simulink model "BimanualHD2LfD"  (R2016b)
settings: Solver=ode1  StartTime=0.0  StopTime=inf  FixedStep=0.002  RelTol=1e-3  EnableMultiTasking=on
undefined symbols (not defined in the file or in its folder): d2r, HIL, qc_get_step_size
libraries: quarc_library x10, simulink_extras x4, dsparch4 x3, simulink x2
(part 1 of 2)
settings Model: SimulationMode=external  ExtModeTrigDuration=120000  Creator=user  LastModifiedBy=Jason
settings SolverCC: PositivePriorityOrder=on
settings DataIOCC: LimitDataPoints=on  SaveFormat=Array  SignalLoggingSaveFormat=ModelDataLogs
settings OptimizationCC: ExpressionDepthLimit=2147483647  LifeSpan=inf
settings DebuggingCC: UnderspecifiedInitializationDetection=Classic  MergeDetectMultiDrivingBlocksExec=none  SolverPrmCheckMsg=warning  FcnCallInpInsideContextMsg=warning  StateNameClashWarn=warning  SFUnexpectedBacktrackingDiag=warning  SFNoUnconditionalDefaultTransitionDiag=warning  SFExecutionAtInitializationDiag=none
settings HardwareCC: ProdBitPerPointer=32  ProdBitPerSizeT=32  ProdBitPerPtrDiffT=32  ProdLargestAtomicFloat=None  ProdIntDivRoundTo=Undefined  ProdEndianess=Unspecified  ProdWordSize=32  ProdHWDeviceType=32-bit Generic
settings ModelReferenceCC: PropagateSignalLabelsOutOfModel=off
settings RTWCC: SystemTargetFile=quarc_windows.tlc  TemplateMakefile=quarc_default_tmf  Description=QUARC Win32 Target
settings STFCustomTargetCC: TargetPreCompLibLocation=C:\PROGRA~2\QUARC\lib\2011b\windows\release  GeneratePreprocessorConditionals=Disable all  CPPClassGenCompliant=on  SystemTargetFile=quarc_windows.tlc
settings GRTTargetCC: TargetPreCompLibLocation=C:\PROGRA~2\QUARC\lib\2011b\windows\release  TargetLangStandard=C89/C90 (ANSI)  ParMdlRefBuildCompliant=off  CompOptLevelCompliant=off  ConcurrentExecutionCompliant=off  GeneratePreprocessorConditionals=Disable all  CombineOutputUpdateFcns=off  MatFileLogging=off  GRTInterface=on  UseToolchainInfoCompliant=off  ExtMode=on  ExtModeMexFile=quarc_comm
settings ConfigComp: CovMetricSettings=dw  CovHtmlReporting=on  CovSaveCumulativeToWorkspaceVar=on  CovSaveSingleToWorkspaceVar=on  CovExternalEMLEnable=off
settings SimEventsCC: propDiagStatOutput=1  propPreventDuplicateEvents=0

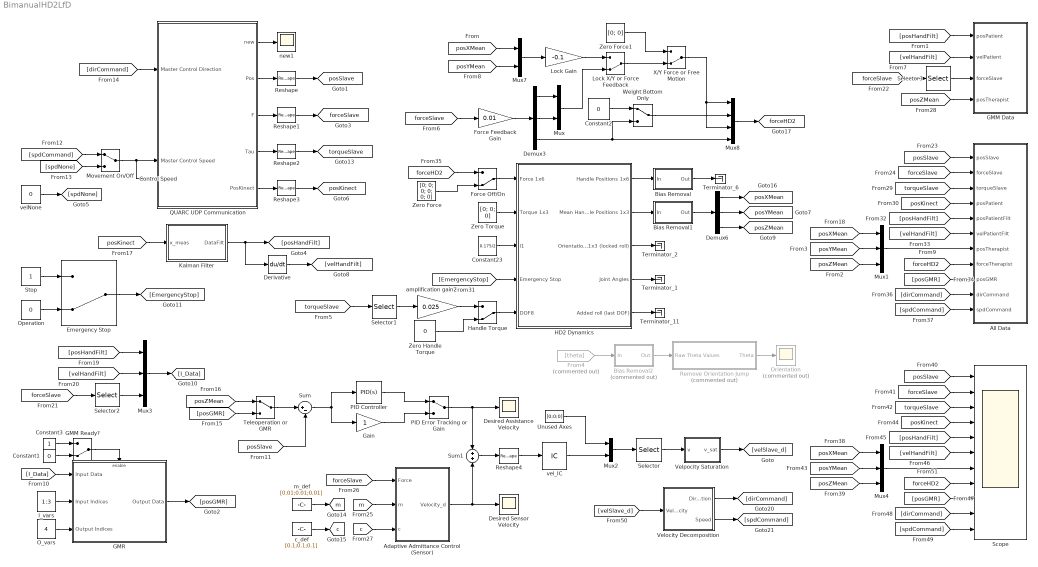
== system BimanualHD2LfD ==
  Adaptive Admittance Control (Sensor) : Subsystem
  All Data : Subsystem  TreatAsAtomicUnit=on
  Bias Removal : Subsystem
  Bias Removal1 : Subsystem
  Bias Removal2 : Subsystem  Commented=on
  Constant1 : Constant  Value=0
  Constant2 : Constant  Value=0
  Constant23 : Constant  Value=0.175/2
  Constant3 : Constant
  Control Speed : Scope
  Demux3 : Demux  Outputs=3
  Demux6 : Demux  Outputs=3
  Derivative : Derivative
  Desired Assistance Velocity : Scope
  Desired Sensor Velocity : Scope
  Emergency Stop : ManualSwitch  CurrentSetting=0
  Force Feedback Gain : Gain  Gain=0.01
  Force Off/On : ManualSwitch  CurrentSetting=0
  From4 : From  Commented=on  GotoTag=theta  TagVisibility=global
  GMM Data : Subsystem  TreatAsAtomicUnit=on
  GMM Ready? : ManualSwitch  CurrentSetting=0
  GMR : Subsystem
  Gain : Gain
  HD2 Dynamics : Subsystem
  Handle Torque : ManualSwitch  CurrentSetting=0
  I_vars : Constant  Value=1:3
  Kalman Filter : MATLAB Function  TreatAsAtomicUnit=on
  Lock Gain : Gain  Gain=-0.1
  Lock X/Y or Force Feedback : ManualSwitch  CurrentSetting=0
  Movement On/Off : ManualSwitch
  Mux : Mux  Inputs=2
  Mux1 : Mux  Inputs=3
  Mux2 : Mux  Inputs=2
  Mux3 : Mux  Inputs=3
  Mux4 : Mux  Inputs=3
  Mux7 : Mux  Inputs=2
  Mux8 : Mux
  O_vars : Constant  Value=4
  Operation : Constant  Value=0
  Orientation : Scope  Commented=on
  PID Controller : simulink/Continuous/PID Controller  Controller=PID  TimeDomain=Continuous-time  SampleTime=-1  IntegratorMethod=Forward Euler  FilterMethod=Forward Euler  Form=Parallel  UseFilter=on  ControllerParametersSource=internal  P=1  I=1  D=0  N=100  InitialConditionSource=internal  InitialConditionForIntegrator=0  InitialConditionForFilter=0  ExternalReset=none  LimitOutput=off  UpperSaturationLimit=inf  LowerSaturationLimit=-inf  LinearizeAsGain=on  AntiWindupMode=none  Kb=1  TrackingMode=off  Kt=1  PParamMin=[]  PParamMax=[]  IParamMin=[]  IParamMax=[]  DParamMin=[]  DParamMax=[]  NParamMin=[]  NParamMax=[]  KbParamMin=[]  KbParamMax=[]  KtParamMin=[]  KtParamMax=[]  POutMin=[]  POutMax=[]  IOutMin=[]  IOutMax=[]  DOutMin=[]  DOutMax=[]  NOutMin=[]  NOutMax=[]  KbOutMin=[]  KbOutMax=[]  KtOutMin=[]  KtOutMax=[]  IntegratorOutMin=[]  IntegratorOutMax=[]  FilterOutMin=[]  FilterOutMax=[]  SumOutMin=[]  SumOutMax=[]  SumI1OutMin=[]  SumI1OutMax=[]  SumI2OutMin=[]  SumI2OutMax=[]  SumI3OutMin=[]  SumI3OutMax=[]  SumDOutMin=[]  SumDOutMax=[]  SaturationOutMin=[]  SaturationOutMax=[]  IntegratorContinuousStateAttributes=''  IntegratorStateMustResolveToSignalObject=off  IntegratorRTWStateStorageClass=Auto  FilterContinuousStateAttributes=''  FilterStateMustResolveToSignalObject=off  FilterRTWStateStorageClass=Auto  DifferentiatorICPrevScaledInput=0  DifferentiatorOutMin=[]  DifferentiatorOutMax=[]
  PID Error Tracking or Gain : ManualSwitch
  QUARC UDP Communication : Subsystem
  Remove Orientation Jump : Subsystem  Commented=on
  Reshape{,1..4} (5 alike) : Reshape  OutputDimensionality=Column vector (2-D)
  Scope : Scope  NumInputPorts=11
  Selector : Selector  InputPortWidth=6  IndexOptions=Index vector (dialog)  Indices=[1 2 6]  OutputSizes=1
  Selector1 : Selector  InputPortWidth=3  IndexOptions=Index vector (dialog)  Indices=[3]  OutputSizes=1
  Selector2 : Selector  InputPortWidth=3  IndexOptions=Index vector (dialog)  Indices=[3]  OutputSizes=1
  Selector3 : Selector  InputPortWidth=3  IndexOptions=Index vector (dialog)  Indices=[3]  OutputSizes=1
  Stop : Constant
  Sum : Sum  Inputs=|+-
  Sum1 : Sum
  Teleoperation or GMR : ManualSwitch
  Terminator_{1..2,6,11} (4 alike) : Terminator
  Unused Axes : Constant  Value=[0;0;0]
  Velocity Decomposition : Subsystem
  Velpocity Saturation : Subsystem
  Weight Bottom Only : ManualSwitch
  X/Y Force or Free Motion : ManualSwitch  CurrentSetting=0
  Zero Force : Constant  Value=[0; 0; 0; 0; 0; 0]
  Zero Force1 : Constant  Value=[0; 0]
  Zero Handle Torque : Constant  Value=0
  Zero Torque : Constant  Value=[0; 0; 0]
  amplification gain2 : Gain  Gain=0.025
  c_def : Constant  Value=[0.1;0.1;0.1]
  m_def : Constant  Value=[0.01;0.01;0.01]
  new1 : Scope
  velNone : Constant  Value=0
  vel_IC : InitialCondition  Value=[0; 0; 0]
  tag scope: c=global, forceHD2=global, forceSlave=global, m=global, posKinect=global, posSlave=global, posXMean=global, posYMean=global, posZMean=global, torqueSlave=global
  wires:
  Zero Torque/1 -> HD2 Dynamics/2(Torque 1x3)
  Constant23/1 -> HD2 Dynamics/3(l1)
  [EmergencyStop] -> HD2 Dynamics/4(Emergency Stop)
  Selector1/1 -> amplification gain2/1
  Handle Torque/1 -> HD2 Dynamics/5(DOF8)
  amplification gain2/1 -> Handle Torque/1
  Zero Handle Torque/1 -> Handle Torque/2
  Demux6/1 -> [posXMean]
  Demux6/2 -> [posYMean]
  Demux6/3 -> [posZMean]
  Force Off/On/1 -> HD2 Dynamics/1(Force 1x6)
  Zero Force/1 -> Force Off/On/2
  HD2 Dynamics/5(Added roll (last DOF)) -> Terminator_11/1
  HD2 Dynamics/4(Joint Angles) -> Terminator_1/1
  HD2 Dynamics/3(Orientation 1x3 (locked roll)) -> Terminator_2/1
  HD2 Dynamics/1(Handle Positions 1x6) -> Bias Removal/1(In)
  Bias Removal/1(Out) -> Terminator_6/1
  [posKinect] -> Kalman Filter/1(x_meas)
  Kalman Filter/1(DataFilt) -> Derivative/1, [posHandFilt]
  HD2 Dynamics/2(Mean Handle Positions 1x3) -> Bias Removal1/1(In)
  Bias Removal1/1(Out) -> Demux6/1
  From4/1 -> Bias Removal2/1(In)
  Bias Removal2/1(Out) -> Remove Orientation Jump/1(Raw Theta Values)
  Remove Orientation Jump/1(Theta) -> Orientation/1
  [forceSlave] -> Force Feedback Gain/1
  Force Feedback Gain/1 -> Demux3/1
  Demux3/1 -> Mux/1
  Demux3/2 -> Mux/2
  Lock X/Y or Force Feedback/1 -> X/Y Force or Free Motion/2
  [posYMean] -> Mux7/2
  [posXMean] -> Mux7/1
  Mux7/1 -> Lock Gain/1
  Mux/1 -> Lock X/Y or Force Feedback/2
  QUARC UDP Communication/1(new) -> new1/1
  QUARC UDP Communication/3(F) -> Reshape1/1
  [dirCommand] -> QUARC UDP Communication/1(Master Control Direction)
  QUARC UDP Communication/2(Pos) -> Reshape/1
  velNone/1 -> [spdNone]
  [spdNone] -> Movement On/Off/2
  [spdCommand] -> Movement On/Off/1
  Reshape1/1 -> [forceSlave]
  Reshape/1 -> [posSlave]
  Reshape2/1 -> [torqueSlave]
  QUARC UDP Communication/5(PosKinect) -> Reshape3/1
  Movement On/Off/1 -> Control Speed/1, QUARC UDP Communication/2(Master Control Speed)
  QUARC UDP Communication/4(Tau) -> Reshape2/1
  [forceSlave] -> Adaptive Admittance Control (Sensor)/1(Force)
  Reshape4/1 -> vel_IC/1
  Sum1/1 -> Reshape4/1
  Adaptive Admittance Control (Sensor)/1(Velocity_d) -> Sum1/2, Desired Sensor Velocity/1
  [m] -> Adaptive Admittance Control (Sensor)/2(m)
  [c] -> Adaptive Admittance Control (Sensor)/3(c)
  PID Error Tracking or Gain/1 -> Sum1/1, Desired Assistance Velocity/1
  Velocity Decomposition/1(Direction) -> [dirCommand]
  Velocity Decomposition/2(Speed) -> [spdCommand]
  [velSlave_d] -> Velocity Decomposition/1(Velocity)
  Velpocity Saturation/1(v_sat) -> [velSlave_d]
  Selector/1 -> Velpocity Saturation/1(v)
  Mux2/1 -> Selector/1
  Unused Axes/1 -> Mux2/1
  vel_IC/1 -> Mux2/2
  Constant2/1 -> Weight Bottom Only/1
  X/Y Force or Free Motion/1 -> Mux8/3, Mux8/1
  Demux3/3 -> Mux8/4, Weight Bottom Only/2
  Weight Bottom Only/1 -> Mux8/2
  Zero Force1/1 -> X/Y Force or Free Motion/1
  Lock Gain/1 -> Lock X/Y or Force Feedback/1
  Mux8/1 -> [forceHD2]
  [forceHD2] -> Force Off/On/1
  I_vars/1 -> GMR/2(Input Indices)
  O_vars/1 -> GMR/3(Output Indices)
  Constant1/1 -> GMM Ready?/2
  Constant3/1 -> GMM Ready?/1
  GMM Ready?/1 -> GMR/Enable
  [I_Data] -> GMR/1(Input Data)
  Reshape3/1 -> [posKinect]
  GMR/1(Output Data) -> [posGMR]
  [posGMR] -> Teleoperation or GMR/2
  [posZMean] -> Teleoperation or GMR/1
  Teleoperation or GMR/1 -> Sum/1
  Sum/1 -> PID Controller/1, Gain/1
  [posSlave] -> Sum/2
  Gain/1 -> PID Error Tracking or Gain/2
  PID Controller/1 -> PID Error Tracking or Gain/1
  [torqueSlave] -> Selector1/1
  Derivative/1 -> [velHandFilt]
  [forceSlave] -> Selector2/1
  [velHandFilt] -> Mux3/2
  Selector2/1 -> Mux3/3
  [posHandFilt] -> Mux3/1
  Mux3/1 -> [I_Data]
  Operation/1 -> Emergency Stop/2
  Stop/1 -> Emergency Stop/1
  Emergency Stop/1 -> [EmergencyStop]
  m_def/1 -> [m]
  c_def/1 -> [c]
  [forceSlave] -> Selector3/1
  Selector3/1 -> GMM Data/3(forceSlave)
  [velHandFilt] -> GMM Data/2(velPatient)
  [posHandFilt] -> GMM Data/1(posPatient)
  [posZMean] -> GMM Data/4(posTherapist)
  [posXMean] -> Mux1/1
  [posYMean] -> Mux1/2
  [posZMean] -> Mux1/3
  [posSlave] -> All Data/1(posSlave)
  [forceSlave] -> All Data/2(forceSlave)
  [torqueSlave] -> All Data/3(torqueSlave)
  [posKinect] -> All Data/4(posPatient)
  [posHandFilt] -> All Data/5(posPatientFilt)
  [velHandFilt] -> All Data/6(velPatientFilt)
  Mux1/1 -> All Data/7(posTherapist)
  [posGMR] -> All Data/9(posGMR)
  [forceHD2] -> All Data/8(forceTherapist)
  [spdCommand] -> All Data/11(spdCommand)
  [dirCommand] -> All Data/10(dirCommand)
  [posXMean] -> Mux4/1
  [posYMean] -> Mux4/2
  [posZMean] -> Mux4/3
  Mux4/1 -> Scope/7
  [posKinect] -> Scope/4
  [velHandFilt] -> Scope/6
  [forceSlave] -> Scope/2
  [posSlave] -> Scope/1
  [torqueSlave] -> Scope/3
  [posHandFilt] -> Scope/5
  [forceHD2] -> Scope/8
  [spdCommand] -> Scope/11
  [dirCommand] -> Scope/10
  [posGMR] -> Scope/9

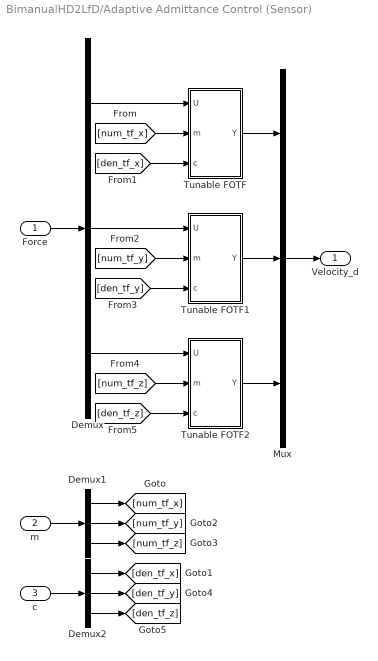
== system BimanualHD2LfD/Adaptive Admittance Control (Sensor) ==
  Force : Inport
  m : Inport  Port=2
  c : Inport  Port=3
  Demux : Demux  Outputs=3
  Demux1 : Demux  Outputs=3
  Demux2 : Demux  Outputs=3
  Mux : Mux  Inputs=3
  Tunable FOTF : Subsystem
  Tunable FOTF1 : Subsystem
  Tunable FOTF2 : Subsystem
  Velocity_d : Outport
  wires:
  Force/1 -> Demux/1
  Mux/1 -> Velocity_d/1
  Tunable FOTF/1(Y) -> Mux/1
  Tunable FOTF1/1(Y) -> Mux/2
  Tunable FOTF2/1(Y) -> Mux/3
  Demux/1 -> Tunable FOTF/1(U)
  Demux/2 -> Tunable FOTF1/1(U)
  Demux/3 -> Tunable FOTF2/1(U)
  c/1 -> Demux2/1
  [num_tf_x] -> Tunable FOTF/2(m)
  [den_tf_x] -> Tunable FOTF/3(c)
  [num_tf_y] -> Tunable FOTF1/2(m)
  [den_tf_y] -> Tunable FOTF1/3(c)
  [num_tf_z] -> Tunable FOTF2/2(m)
  [den_tf_z] -> Tunable FOTF2/3(c)
  Demux1/1 -> [num_tf_x]
  Demux1/2 -> [num_tf_y]
  Demux1/3 -> [num_tf_z]
  Demux2/1 -> [den_tf_x]
  Demux2/2 -> [den_tf_y]
  Demux2/3 -> [den_tf_z]
  m/1 -> Demux1/1

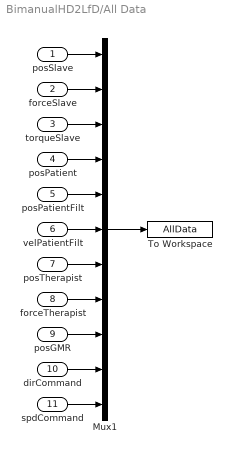
== system BimanualHD2LfD/All Data ==
  posSlave : Inport
  forceSlave : Inport  Port=2
  torqueSlave : Inport  Port=3
  posPatient : Inport  Port=4
  posPatientFilt : Inport  Port=5
  velPatientFilt : Inport  Port=6
  posTherapist : Inport  Port=7
  forceTherapist : Inport  Port=8
  posGMR : Inport  Port=9
  dirCommand : Inport  Port=10
  spdCommand : Inport  Port=11
  Mux1 : Mux  Inputs=11
  To Workspace : ToWorkspace  VariableName=AllData  SaveFormat=Structure With Time  SampleTime=-1
  wires:
  Mux1/1 -> To Workspace/1
  posSlave/1 -> Mux1/1
  forceSlave/1 -> Mux1/2
  torqueSlave/1 -> Mux1/3
  posPatient/1 -> Mux1/4
  velPatientFilt/1 -> Mux1/6
  posPatientFilt/1 -> Mux1/5
  posTherapist/1 -> Mux1/7
  spdCommand/1 -> Mux1/11
  forceTherapist/1 -> Mux1/8
  posGMR/1 -> Mux1/9
  dirCommand/1 -> Mux1/10

== system BimanualHD2LfD/Bias Removal ==
  In : Inport
  Latch : Subsystem
  Sum1 : Sum  Inputs=|+-
  Out : Outport
  wires:
  In/1 -> Sum1/1, Latch/1(x)
  Latch/1(x_target) -> Sum1/2
  Sum1/1 -> Out/1

== system BimanualHD2LfD/Bias Removal1 ==
  In : Inport
  Latch : Subsystem
  Sum1 : Sum  Inputs=|+-
  Out : Outport
  wires:
  In/1 -> Sum1/1, Latch/1(x)
  Latch/1(x_target) -> Sum1/2
  Sum1/1 -> Out/1

== system BimanualHD2LfD/Bias Removal2 ==
  In : Inport
  Latch : Subsystem
  Sum1 : Sum  Inputs=|+-
  Out : Outport
  wires:
  In/1 -> Sum1/1, Latch/1(x)
  Latch/1(x_target) -> Sum1/2
  Sum1/1 -> Out/1

== system BimanualHD2LfD/GMM Data ==
  posPatient : Inport
  velPatient : Inport  Port=2
  forceSlave : Inport  Port=3
  posTherapist : Inport  Port=4
  Mux1 : Mux
  To Workspace : ToWorkspace  VariableName=GMMData  SaveFormat=Structure With Time  SampleTime=-1
  wires:
  Mux1/1 -> To Workspace/1
  posPatient/1 -> Mux1/1
  velPatient/1 -> Mux1/2
  forceSlave/1 -> Mux1/3
  posTherapist/1 -> Mux1/4

== system BimanualHD2LfD/GMR ==
  Input Data : Inport
  Input Indices : Inport  Port=2
  Output Indices : Inport  Port=3
  Enable : EnablePort
  MATLAB Function : MATLAB Function  TreatAsAtomicUnit=on
  Terminator : Terminator
  Output Data : Outport
  wires:
  Output Indices/1 -> MATLAB Function/3(O_vars)
  Input Indices/1 -> MATLAB Function/2(I_vars)
  Input Data/1 -> MATLAB Function/1(data)
  MATLAB Function/1(outputs) -> Output Data/1
  MATLAB Function/2(output_var) -> Terminator/1

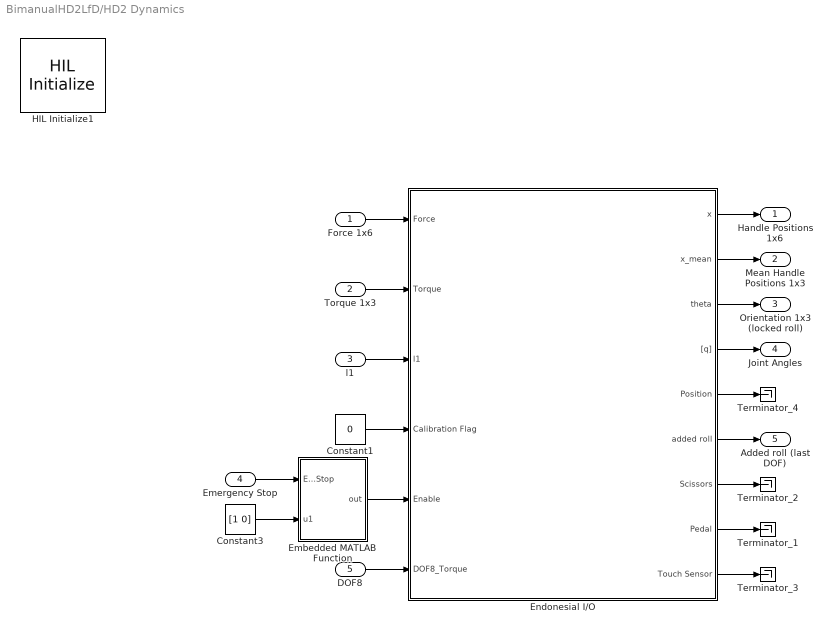
== system BimanualHD2LfD/HD2 Dynamics ==
  Force 1x6 : Inport
  Torque 1x3 : Inport  Port=2
  l1 : Inport  Port=3
  Emergency Stop : Inport  Port=4
  DOF8 : Inport  Port=5
  Constant1 : Constant  Value=0
  Constant3 : Constant  Value=[1 0]
  Embedded MATLAB Function : MATLAB Function  TreatAsAtomicUnit=on
  Endonesial I/O : Subsystem
  HIL Initialize1 : quarc_library/Data Acquisition/Generic/Configuration/HIL Initialize  Priority=0  object_name=HIL-1  board_type=qpid_e  board_number=0  board_options=enc0_dir=0;enc0_filter=1;enc0_a=1;enc0_b=1;enc0_z=0;enc0_reload=0;enc1_dir=0;enc1_filter=1;enc1_a=1;enc1_b=1;enc1_z=0;enc1_reload=0;enc2_dir=0;enc2_filter=1;enc2_a=1;enc2_b=1;enc2_z=0;enc2_reload=0;enc3_dir=0;enc3_filter=1;enc3_a=1;enc3_b=1;enc3_z=0;enc3_reload=0;enc4_dir=0;enc4_filter=1;enc4_a=1;enc4_b=1;enc4_z=0;enc4_reload=0;enc5_dir=0;enc5_filter=1;enc5_a=1;enc5_b=1;enc5_z=0;enc5_reload=0;enc6_dir=0;enc6_filter=1;enc6_a=1;enc6_b=1;enc6_z=0;enc6_reload=0;enc7_dir=0;enc7_filter=1;enc7_a=1;enc7_b=1;enc7_z=0;enc7_reload=0;ext_int_polarity=0;fuse_polarity=0;convert_polarity=0;watchdog_polarity=0;ext_int_watchdog=0;fuse_watchdog=0;trig1_watchdog=0;watchdog_to_trig1=0;watchdog_to_trig2=0;counter_to_trig0=0;trigger_adcs=0;latch_on_adc=0;pwm_immediate=0  exclusive=off  active=on  hardware_clocks=[0:16]  clock_modes=[]  initial_clock_frequencies=[]  set_clock_params_at_start=off  set_clock_params_at_switch_in=off  set_clock_frequencies_at_start=off  set_clock_frequencies_at_switch_in=off  analog_input_channels=[0:7]  analog_input_maximums=10  analog_input_minimums=-10  set_analog_input_params_at_start=off  set_analog_input_params_at_switch_in=off  analog_output_channels=[0:7]  analog_output_maximums=10  analog_output_minimums=-10  initial_analog_outputs=[0]  final_analog_outputs=[0]  watchdog_analog_outputs=0  set_analog_output_params_at_start=off  set_analog_output_params_at_switch_in=off  set_analog_outputs_at_start=on  set_analog_outputs_at_switch_in=off  set_analog_outputs_at_terminate=on  set_analog_outputs_at_switch_out=off  set_analog_outputs_on_watchdog=off  digital_input_channels=[]  digital_output_channels=[9 10]  digital_output_configuration=[]  initial_digital_outputs=[1 1]  final_digital_outputs=[1 1]  watchdog_digital_outputs=[2]  set_digital_output_params_at_start=off  set_digital_output_params_at_switch_in=off  set_digital_outputs_at_start=on  set_digital_outputs_at_switch_in=off  set_digital_outputs_at_terminate=on  set_digital_outputs_at_switch_out=off  set_digital_outputs_on_watchdog=off  encoder_channels=[0:7]  quadrature=[4]  encoder_filter_frequency=40e6/1  initial_encoder_counts=[0]  set_encoder_params_at_start=on  set_encoder_params_at_switch_in=off  set_encoder_counts_at_start=off  set_encoder_counts_at_switch_in=off  pwm_channels=[0:7]  pwm_modes=0  pwm_frequency=40e6/4096  pwm_configuration=[0]  pwm_alignment=[0]  pwm_polarity=[1]  pwm_leading_deadband=[0]  pwm_trailing_deadband=[0]  initial_pwm_outputs=[0]  final_pwm_outputs=[0]  watchdog_pwm_outputs=[0]  set_pwm_params_at_start=on  set_pwm_params_at_switch_in=off  set_pwm_outputs_at_start=on  set_pwm_outputs_at_switch_in=off  set_pwm_outputs_at_terminate=on  set_pwm_outputs_at_switch_out=off  set_pwm_outputs_on_watchdog=off  other_output_channels=[]  initial_other_outputs=[]  final_other_outputs=[]  watchdog_other_outputs=[]  set_other_outputs_at_start=off  set_other_outputs_at_switch_in=off  set_other_outputs_at_terminate=off  set_other_outputs_at_switch_out=off  set_other_outputs_on_watchdog=off
  Terminator_{1..4} (4 alike) : Terminator
  Handle Positions 1x6 : Outport
  Mean Handle Positions 1x3 : Outport  Port=2
  Orientation 1x3 (locked roll) : Outport  Port=3
  Joint Angles : Outport  Port=4
  Added roll (last DOF) : Outport  Port=5
  wires:
  Endonesial I/O/2(x_mean) -> Mean Handle Positions 1x3/1
  Constant1/1 -> Endonesial I/O/4(Calibration Flag)
  Torque 1x3/1 -> Endonesial I/O/2(Torque)
  Emergency Stop/1 -> Embedded MATLAB Function/1(EmergStop)
  Constant3/1 -> Embedded MATLAB Function/2(u1)
  Embedded MATLAB Function/1(out) -> Endonesial I/O/5(Enable)
  Endonesial I/O/1(x) -> Handle Positions 1x6/1
  Force 1x6/1 -> Endonesial I/O/1(Force)
  Endonesial I/O/3(theta) -> Orientation 1x3 (locked roll)/1
  Endonesial I/O/4("[q]") -> Joint Angles/1
  Endonesial I/O/5(Position) -> Terminator_4/1
  Endonesial I/O/6(added roll) -> Added roll (last DOF)/1
  Endonesial I/O/8(Pedal) -> Terminator_1/1
  Endonesial I/O/7(Scissors) -> Terminator_2/1
  Endonesial I/O/9(Touch Sensor) -> Terminator_3/1
  l1/1 -> Endonesial I/O/3(l1)
  DOF8/1 -> Endonesial I/O/6(DOF8_Torque)

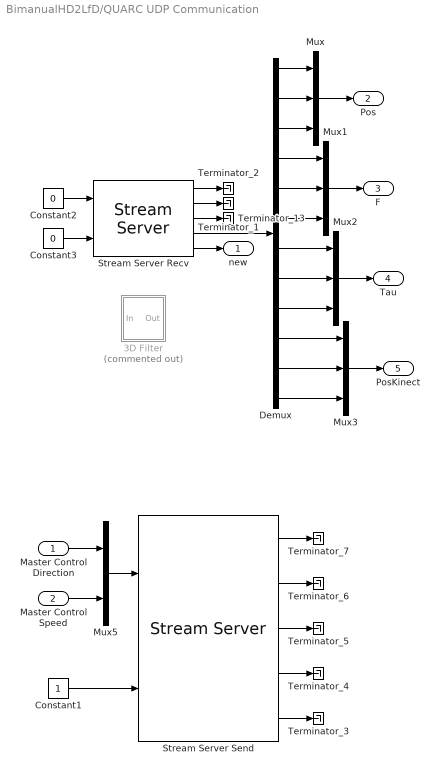
== system BimanualHD2LfD/QUARC UDP Communication ==
  Master Control Direction : Inport
  Master Control Speed : Inport  Port=2
  3D Filter : Subsystem  Commented=on
  Constant1 : Constant
  Constant2 : Constant  Value=0
  Constant3 : Constant  Value=0
  Demux : Demux  Outputs=12
  Mux{,1..3} (4 alike) : Mux  Inputs=3
  Mux5 : Mux  Inputs=2
  Stream Server Recv : quarc_library/Communications/Basic/Stream Server  uri_source=Specify via dialog (do not evaluate)  uri=shmem://UDPmem_recv:2?local=yes  apply_uri_to_all_configs=on  send_buffer_size=1460  receive_buffer_size=1460  byte_order=little endian (Intel - LSB first)  optimization=Minimum latency  send_options=Send most recent data  receive_options=Receive most recent data  default_value=[0 0 0 0 0 0 0 0 0 0 0 0 0 0 0]  sample_time=qc_get_step_size  active=on  implementation=Use blocking I/O in a separate thread  send_fifo_size=1000  receive_fifo_size=1000  send_priority=0  receive_priority=0  send_dimensions=off  receive_dimensions=off  max_dimensions=-1  data_type=Inherited via back propagation  type_expr=BusObject
      settings: AttributesFormatString="\"shmem://UDPmem_recv:2?local=yes\""
  Stream Server Send : quarc_library/Communications/Basic/Stream Server  uri_source=Specify via dialog (do not evaluate)  uri=shmem://UDPmem_send:1?local=yes  apply_uri_to_all_configs=on  send_buffer_size=1460  receive_buffer_size=1460  byte_order=little endian (Intel - LSB first)  optimization=Minimum latency  send_options=Send most recent data  receive_options=Receive most recent data  default_value=[0 0 0 0]  sample_time=qc_get_step_size  active=on  implementation=Use blocking I/O in a separate thread  send_fifo_size=1000  receive_fifo_size=1000  send_priority=0  receive_priority=0  send_dimensions=off  receive_dimensions=off  max_dimensions=-1  data_type=Inherited via back propagation  type_expr=BusObject
      settings: AttributesFormatString="\"shmem://UDPmem_send:1?local=yes\""
  Terminator_{1..7,13} (8 alike) : Terminator
  new : Outport
  Pos : Outport  Port=2
  F : Outport  Port=3
  Tau : Outport  Port=4
  PosKinect : Outport  Port=5
  wires:
  Constant2/1 -> Stream Server Recv/1
  Constant1/1 -> Stream Server Send/2
  Stream Server Send/1 -> Terminator_7/1
  Stream Server Send/2 -> Terminator_6/1
  Stream Server Send/3 -> Terminator_5/1
  Stream Server Send/4 -> Terminator_4/1
  Stream Server Send/5 -> Terminator_3/1
  Constant3/1 -> Stream Server Recv/2
  Stream Server Recv/1 -> Terminator_2/1
  Stream Server Recv/2 -> Terminator_1/1
  Stream Server Recv/3 -> Terminator_13/1
  Stream Server Recv/5 -> new/1
  Stream Server Recv/4 -> Demux/1
  Mux/1 -> Pos/1
  Mux2/1 -> Tau/1
  Demux/7 -> Mux2/1
  Demux/8 -> Mux2/2
  Demux/9 -> Mux2/3
  Demux/4 -> Mux1/1
  Demux/5 -> Mux1/2
  Demux/6 -> Mux1/3
  Demux/1 -> Mux/1
  Demux/2 -> Mux/2
  Demux/3 -> Mux/3
  Mux5/1 -> Stream Server Send/1
  Master Control Direction/1 -> Mux5/1
  Master Control Speed/1 -> Mux5/2
  Mux1/1 -> F/1
  Mux3/1 -> PosKinect/1
  Demux/10 -> Mux3/1
  Demux/11 -> Mux3/2
  Demux/12 -> Mux3/3

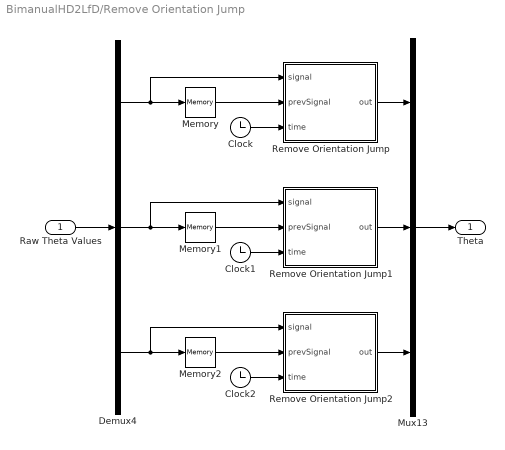
== system BimanualHD2LfD/Remove Orientation Jump ==
  Raw Theta Values : Inport
  Clock : Clock
  Clock1 : Clock
  Clock2 : Clock
  Demux4 : Demux  Outputs=3
  Memory : Memory
  Memory1 : Memory
  Memory2 : Memory
  Mux13 : Mux  Inputs=3
  Remove Orientation Jump : MATLAB Function  TreatAsAtomicUnit=on
  Remove Orientation Jump1 : MATLAB Function  TreatAsAtomicUnit=on
  Remove Orientation Jump2 : MATLAB Function  TreatAsAtomicUnit=on
  Theta : Outport
  wires:
  Demux4/1 -> Remove Orientation Jump/1(signal), Memory/1
  Memory/1 -> Remove Orientation Jump/2(prevSignal)
  Clock/1 -> Remove Orientation Jump/3(time)
  Remove Orientation Jump/1(out) -> Mux13/1
  Mux13/1 -> Theta/1
  Raw Theta Values/1 -> Demux4/1
  Demux4/2 -> Remove Orientation Jump1/1(signal), Memory1/1
  Memory1/1 -> Remove Orientation Jump1/2(prevSignal)
  Clock1/1 -> Remove Orientation Jump1/3(time)
  Remove Orientation Jump1/1(out) -> Mux13/2
  Demux4/3 -> Remove Orientation Jump2/1(signal), Memory2/1
  Memory2/1 -> Remove Orientation Jump2/2(prevSignal)
  Clock2/1 -> Remove Orientation Jump2/3(time)
  Remove Orientation Jump2/1(out) -> Mux13/3

== system BimanualHD2LfD/Velocity Decomposition ==
  Velocity : Inport
  MATLAB Function : MATLAB Function  TreatAsAtomicUnit=on
  Direction : Outport
  Speed : Outport  Port=2
  wires:
  Velocity/1 -> MATLAB Function/1(velDes)
  MATLAB Function/1(dirDes) -> Direction/1
  MATLAB Function/2(spdDes) -> Speed/1

== system BimanualHD2LfD/Velpocity Saturation ==
  v : Inport
  MATLAB Function : MATLAB Function  TreatAsAtomicUnit=on
  v_sat : Outport
  wires:
  v/1 -> MATLAB Function/1(v)
  MATLAB Function/1(v_sat) -> v_sat/1

== system BimanualHD2LfD/Adaptive Admittance Control (Sensor)/Tunable FOTF ==
  U : Inport
  m : Inport  Port=2
  c : Inport  Port=3
  Divide1 : Product  Inputs=/**
  Integrator1 : Integrator
  Integrator2 : Integrator
  Product : Product  Inputs=*/
  Sum : Sum  Inputs=|+-
  Y : Outport
  wires:
  U/1 -> Integrator1/1
  Integrator1/1 -> Product/1
  m/1 -> Divide1/1, Product/2
  Product/1 -> Sum/1
  Sum/1 -> Integrator2/1, Y/1
  c/1 -> Divide1/2
  Divide1/1 -> Sum/2
  Integrator2/1 -> Divide1/3

== system BimanualHD2LfD/Adaptive Admittance Control (Sensor)/Tunable FOTF1 ==
  U : Inport
  m : Inport  Port=2
  c : Inport  Port=3
  Divide1 : Product  Inputs=/**
  Integrator1 : Integrator
  Integrator2 : Integrator
  Product : Product  Inputs=*/
  Sum : Sum  Inputs=|+-
  Y : Outport
  wires:
  U/1 -> Integrator1/1
  Integrator1/1 -> Product/1
  m/1 -> Divide1/1, Product/2
  Product/1 -> Sum/1
  Sum/1 -> Integrator2/1, Y/1
  c/1 -> Divide1/2
  Divide1/1 -> Sum/2
  Integrator2/1 -> Divide1/3

== system BimanualHD2LfD/Adaptive Admittance Control (Sensor)/Tunable FOTF2 ==
  U : Inport
  m : Inport  Port=2
  c : Inport  Port=3
  Divide1 : Product  Inputs=/**
  Integrator1 : Integrator
  Integrator2 : Integrator
  Product : Product  Inputs=*/
  Sum : Sum  Inputs=|+-
  Y : Outport
  wires:
  U/1 -> Integrator1/1
  Integrator1/1 -> Product/1
  m/1 -> Divide1/1, Product/2
  Product/1 -> Sum/1
  Sum/1 -> Integrator2/1, Y/1
  c/1 -> Divide1/2
  Divide1/1 -> Sum/2
  Integrator2/1 -> Divide1/3

== system BimanualHD2LfD/Bias Removal/Latch ==
  x : Inport
  Clock : Clock
  Constant1 : Constant
  Constant2 : Constant  Value=0
  Latch Input : Subsystem  TreatAsAtomicUnit=on
  Switch1 : Switch  Threshold=0.0001
  Terminator_13 : Terminator
  x_target : Outport
  wires:
  Latch Input/1(Latch) -> x_target/1
  x/1 -> Latch Input/1(Input)
  Switch1/1 -> Latch Input/Trigger
  Constant1/1 -> Switch1/1
  Clock/1 -> Switch1/2
  Constant2/1 -> Switch1/3
  Latch Input/2(Executed) -> Terminator_13/1

== system BimanualHD2LfD/Bias Removal1/Latch ==
  x : Inport
  Clock : Clock
  Constant1 : Constant
  Constant2 : Constant  Value=0
  Latch Input : Subsystem  TreatAsAtomicUnit=on
  Switch1 : Switch  Threshold=0.0001
  Terminator_13 : Terminator
  x_target : Outport
  wires:
  Latch Input/1(Latch) -> x_target/1
  x/1 -> Latch Input/1(Input)
  Switch1/1 -> Latch Input/Trigger
  Constant1/1 -> Switch1/1
  Clock/1 -> Switch1/2
  Constant2/1 -> Switch1/3
  Latch Input/2(Executed) -> Terminator_13/1

== system BimanualHD2LfD/Bias Removal2/Latch ==
  x : Inport
  Clock : Clock
  Constant1 : Constant
  Constant2 : Constant  Value=0
  Latch Input : Subsystem  TreatAsAtomicUnit=on
  Switch1 : Switch  Threshold=0.0001
  Terminator_13 : Terminator
  x_target : Outport
  wires:
  Latch Input/1(Latch) -> x_target/1
  x/1 -> Latch Input/1(Input)
  Switch1/1 -> Latch Input/Trigger
  Constant1/1 -> Switch1/1
  Clock/1 -> Switch1/2
  Constant2/1 -> Switch1/3
  Latch Input/2(Executed) -> Terminator_13/1

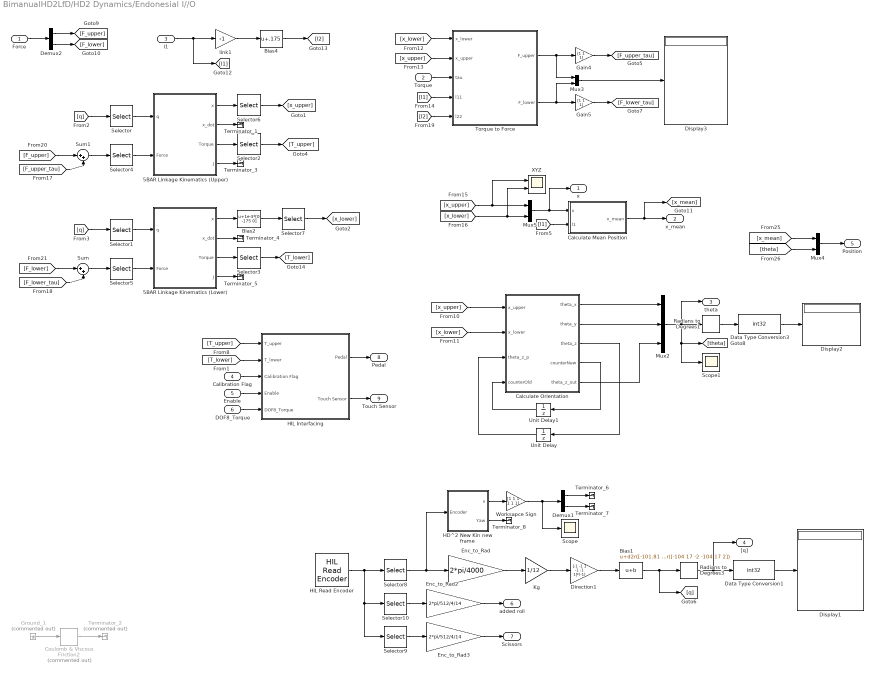
== system BimanualHD2LfD/HD2 Dynamics/Endonesial I//O ==
  Force : Inport
  Torque : Inport  Port=2
  l1 : Inport  Port=3
  Calibration Flag : Inport  Port=4
  Enable : Inport  Port=5
  DOF8_Torque : Inport  Port=6
  5BAR Linkage Kinematics (Lower) : Subsystem  AncestorBlock=quanser_tunable_functions/Kinematics/5BAR Linkage Kinematics
  5BAR Linkage Kinematics (Upper) : Subsystem  AncestorBlock=quanser_tunable_functions/Kinematics/5BAR Linkage Kinematics
  Bias1 : Bias  Bias=d2r([-101.81 13.31 -4.4 -101.3 13.42 9.64])%d2r([-104 17 -2 -104 17 2])
  Bias2 : Bias  Bias=1e-3*[0 -175 0]
  Bias4 : Bias  Bias=.175
  Calculate Mean Position : MATLAB Function  TreatAsAtomicUnit=on
  Calculate Orientation : MATLAB Function  TreatAsAtomicUnit=on
  Coulomb & Viscous Friction2 : simulink/Discontinuities/Coulomb & Viscous Friction  Commented=on  offset=0.01  gain=1
  Data Type Conversion1 : DataTypeConversion  OutDataTypeStr=int32
  Data Type Conversion3 : DataTypeConversion  OutDataTypeStr=int32
  Demux1 : Demux  Outputs=[3 3]
  Demux2 : Demux  Outputs=[3 3]
  Direction1 : Gain  Gain=[-1 -1 1 -1 -1 1]*(-1)
  Display1 : Display
      settings: Decimation=100
  Display2 : Display
      settings: Decimation=100
  Display3 : Display
      settings: Decimation=1000
  Enc_to_Rad : Gain  Gain=2*pi/4000
  Enc_to_Rad2 : Gain  Gain=2*pi/512/4/14
  Enc_to_Rad3 : Gain  Gain=2*pi/512/4/14
  Gain4 : Gain  Gain=[1 1 1]
  Gain5 : Gain  Gain=[1 1 1]
  Ground_1 : Ground  Commented=on
  HD^2 New Kin new frame : Subsystem
  HIL Interfacing : Subsystem
  HIL Read Encoder : quarc_library/Data Acquisition/Generic/Immediate I//O/HIL Read Encoder  object_name=HIL-1  channels=0:7  sample_time=qc_get_step_size  active=on  vector_output=on  data_type_mode=Inherit via back propagation  data_type=double
  Kg : Gain  Gain=1/12
  Mux2 : Mux  Inputs=3
  Mux3 : Mux  Inputs=2
  Mux4 : Mux  Inputs=2
  Mux5 : Mux  Inputs=[3 3]
  Radians to Degrees1 : simulink_extras/Transformations/Radians to Degrees
  Radians to Degrees3 : simulink_extras/Transformations/Radians to Degrees
  Scope : Scope
  Scope1 : Scope
  Selector : Selector  InputPortWidth=6  IndexOptions=Index vector (dialog)  Indices=[3 2 1]  OutputSizes=1
  Selector1 : Selector  InputPortWidth=6  IndexOptions=Index vector (dialog)  Indices=[6 5 4]  OutputSizes=1
  Selector10 : Selector  InputPortWidth=8  IndexOptions=Index vector (dialog)  Indices=7  OutputSizes=1
  Selector2 : Selector  InputPortWidth=3  IndexOptions=Index vector (dialog)  Indices=[3 2 1]  OutputSizes=1
  Selector3 : Selector  InputPortWidth=3  IndexOptions=Index vector (dialog)  Indices=[3 2 1]  OutputSizes=1
  Selector4 : Selector  InputPortWidth=3  IndexOptions=Index vector (dialog)  Indices=[2 3 1]  OutputSizes=1
  Selector5 : Selector  InputPortWidth=3  IndexOptions=Index vector (dialog)  Indices=[2 3 1]  OutputSizes=1
  Selector6 : Selector  InputPortWidth=3  IndexOptions=Index vector (dialog)  Indices=[3 1 2]  OutputSizes=1
  Selector7 : Selector  InputPortWidth=3  IndexOptions=Index vector (dialog)  Indices=[3 1 2]  OutputSizes=1
  Selector8 : Selector  InputPortWidth=8  IndexOptions=Index vector (dialog)  Indices=[1:6]  OutputSizes=1
  Selector9 : Selector  InputPortWidth=8  IndexOptions=Index vector (dialog)  Indices=8  OutputSizes=1
  Sum : Sum  Inputs=|++
  Sum1 : Sum  Inputs=|++
  Terminator_{1,3..8} (7 alike) : Terminator
  Terminator_2 : Terminator  Commented=on
  Torque to Force : MATLAB Function  TreatAsAtomicUnit=on
  Unit Delay : UnitDelay  SampleTime=-1
  Unit Delay1 : UnitDelay  SampleTime=-1
  Worksapce Sign : Gain  Gain=[1 1 1 1 1 1]
  XYZ : Scope  NumInputPorts=2
  link1 : Gain  Gain=-1
  x : Outport
  x_mean : Outport  Port=2
  theta : Outport  Port=3
  "[q]" : Outport  Port=4
  Position : Outport  Port=5
  added roll : Outport  Port=6
  Scissors : Outport  Port=7
  Pedal : Outport  Port=8
  Touch Sensor : Outport  Port=9
  wires:
  Data Type Conversion1/1 -> Display1/1
  Radians to Degrees3/1 -> "[q]"/1, Data Type Conversion1/1
  Enc_to_Rad2/1 -> added roll/1
  Selector10/1 -> Enc_to_Rad2/1
  5BAR Linkage Kinematics (Upper)/1(x) -> Selector6/1
  Bias2/1 -> Selector7/1
  Selector6/1 -> [x_upper]
  Selector7/1 -> [x_lower]
  [F_lower_tau] -> Sum/2
  [F_lower] -> Sum/1
  [F_upper_tau] -> Sum1/2
  [F_upper] -> Sum1/1
  5BAR Linkage Kinematics (Lower)/4(J) -> Terminator_5/1
  5BAR Linkage Kinematics (Lower)/2(x_dot) -> Terminator_4/1
  5BAR Linkage Kinematics (Upper)/4(J) -> Terminator_3/1
  5BAR Linkage Kinematics (Upper)/2(x_dot) -> Terminator_1/1
  Selector5/1 -> 5BAR Linkage Kinematics (Lower)/2(Force)
  Selector4/1 -> 5BAR Linkage Kinematics (Upper)/2(Force)
  Sum1/1 -> Selector4/1
  5BAR Linkage Kinematics (Lower)/3(Torque) -> Selector3/1
  Selector3/1 -> [T_lower]
  Selector2/1 -> [T_upper]
  5BAR Linkage Kinematics (Upper)/3(Torque) -> Selector2/1
  5BAR Linkage Kinematics (Lower)/1(x) -> Bias2/1
  Sum/1 -> Selector5/1
  [q] -> Selector1/1
  Selector1/1 -> 5BAR Linkage Kinematics (Lower)/1(q)
  Selector/1 -> 5BAR Linkage Kinematics (Upper)/1(q)
  [q] -> Selector/1
  Coulomb & Viscous Friction2/1 -> Terminator_2/1
  Ground_1/1 -> Coulomb & Viscous Friction2/1
  Mux4/1 -> Position/1
  [theta] -> Mux4/2
  [x_mean] -> Mux4/1
  Enable/1 -> HIL Interfacing/4(Enable)
  HIL Interfacing/2("Touch Sensor ") -> Touch Sensor/1
  HIL Interfacing/1(Pedal) -> Pedal/1
  Calibration Flag/1 -> HIL Interfacing/3(Calibration Flag)
  [T_lower] -> HIL Interfacing/2(T_lower)
  [T_upper] -> HIL Interfacing/1(T_upper)
  Mux2/1 -> Scope1/1, [theta], Radians to Degrees1/1, theta/1
  Calculate Orientation/3(theta_z) -> Unit Delay/1
  HD^2 New Kin new frame/1(x) -> Worksapce Sign/1
  [l2] -> Torque to Force/5(l22)
  [l1] -> Torque to Force/4(l11)
  [l1] -> Calculate Mean Position/2(l1)
  Mux5/1 -> Calculate Mean Position/1(x), x/1
  Calculate Mean Position/1(x_mean) -> x_mean/1, [x_mean]
  [x_lower] -> XYZ/2, Mux5/2
  [x_upper] -> Mux5/1, XYZ/1
  Bias4/1 -> [l2]
  link1/1 -> Bias4/1
  l1/1 -> [l1], link1/1
  Enc_to_Rad3/1 -> Scissors/1
  Selector9/1 -> Enc_to_Rad3/1
  Selector8/1 -> Enc_to_Rad/1, HD^2 New Kin new frame/1(Encoder)
  Worksapce Sign/1 -> Scope/1, Demux1/1
  Gain5/1 -> [F_lower_tau]
  Gain4/1 -> [F_upper_tau]
  Torque/1 -> Torque to Force/3(tau)
  Mux3/1 -> Display3/1
  Torque to Force/2(F_lower) -> Gain5/1, Mux3/2
  Torque to Force/1(F_upper) -> Gain4/1, Mux3/1
  [x_upper] -> Torque to Force/2(x_upper)
  [x_lower] -> Torque to Force/1(x_lower)
  Calculate Orientation/2(theta_y) -> Mux2/2
  Data Type Conversion3/1 -> Display2/1
  Radians to Degrees1/1 -> Data Type Conversion3/1
  Calculate Orientation/1(theta_x) -> Mux2/1
  [x_lower] -> Calculate Orientation/2(x_lower)
  [x_upper] -> Calculate Orientation/1(x_upper)
  Bias1/1 -> Radians to Degrees3/1, [q]
  Kg/1 -> Direction1/1
  Enc_to_Rad/1 -> Kg/1
  HIL Read Encoder/1 -> Selector10/1, Selector9/1, Selector8/1
  Direction1/1 -> Bias1/1
  Unit Delay/1 -> Calculate Orientation/3(theta_z_p)
  Calculate Orientation/4(counterNew) -> Unit Delay1/1
  Unit Delay1/1 -> Calculate Orientation/4(counterOld)
  Calculate Orientation/5(theta_z_out) -> Mux2/3
  DOF8_Torque/1 -> HIL Interfacing/5(DOF8_Torque)
  Demux1/2 -> Terminator_7/1
  Demux1/1 -> Terminator_6/1
  HD^2 New Kin new frame/2(Yaw) -> Terminator_8/1
  Force/1 -> Demux2/1
  Demux2/1 -> [F_upper]
  Demux2/2 -> [F_lower]

== system BimanualHD2LfD/QUARC UDP Communication/3D Filter ==
  In : Inport
  Analog Filter Design : dsparch4/Analog Filter Design  method=Butterworth  filttype=Lowpass  N=3  Wlo=30  Whi=80  Rp=2  Rs=40
  Analog Filter Design1 : dsparch4/Analog Filter Design  method=Butterworth  filttype=Lowpass  N=3  Wlo=30  Whi=80  Rp=2  Rs=40
  Analog Filter Design2 : dsparch4/Analog Filter Design  method=Butterworth  filttype=Lowpass  N=3  Wlo=30  Whi=80  Rp=2  Rs=40
  Demux : Demux  Outputs=3
  Mux : Mux  Inputs=3
  Out : Outport
  wires:
  In/1 -> Demux/1
  Mux/1 -> Out/1
  Demux/1 -> Analog Filter Design/1
  Demux/2 -> Analog Filter Design1/1
  Demux/3 -> Analog Filter Design2/1
  Analog Filter Design2/1 -> Mux/3
  Analog Filter Design1/1 -> Mux/2
  Analog Filter Design/1 -> Mux/1

== system BimanualHD2LfD/Bias Removal/Latch/Latch Input ==
  Input : Inport
  Trigger : TriggerPort  VariantControl=Variant
  Constant : Constant
  Latch : Outport
  Executed : Outport  Port=2
  wires:
  Input/1 -> Latch/1
  Constant/1 -> Executed/1

== system BimanualHD2LfD/Bias Removal1/Latch/Latch Input ==
  Input : Inport
  Trigger : TriggerPort  VariantControl=Variant
  Constant : Constant
  Latch : Outport
  Executed : Outport  Port=2
  wires:
  Input/1 -> Latch/1
  Constant/1 -> Executed/1

== system BimanualHD2LfD/Bias Removal2/Latch/Latch Input ==
  Input : Inport
  Trigger : TriggerPort  VariantControl=Variant
  Constant : Constant
  Latch : Outport
  Executed : Outport  Port=2
  wires:
  Input/1 -> Latch/1
  Constant/1 -> Executed/1

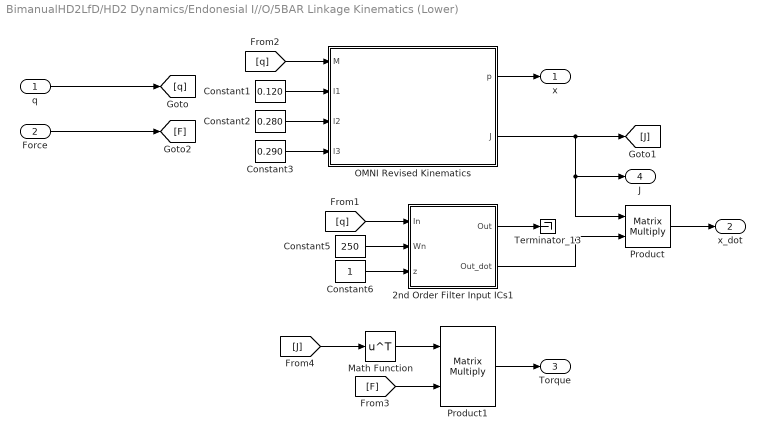
== system BimanualHD2LfD/HD2 Dynamics/Endonesial I//O/5BAR Linkage Kinematics (Lower) ==
  q : Inport
  Force : Inport  Port=2
  2nd Order Filter Input ICs1 : Subsystem
  Constant1 : Constant  Value=0.120
  Constant2 : Constant  Value=0.280
  Constant3 : Constant  Value=0.290
  Constant5 : Constant  Value=250
  Constant6 : Constant
  Math Function : Math  Operator=transpose  SaturateOnIntegerOverflow=on
  OMNI Revised Kinematics : MATLAB Function  TreatAsAtomicUnit=on
  Product : Product  Multiplication=Matrix(*)  RndMeth=Zero
  Product1 : Product  Multiplication=Matrix(*)  RndMeth=Zero
  Terminator_13 : Terminator
  x : Outport
  x_dot : Outport  Port=2
  Torque : Outport  Port=3
  J : Outport  Port=4
  wires:
  Math Function/1 -> Product1/1
  Product1/1 -> Torque/1
  [F] -> Product1/2
  [J] -> Math Function/1
  Force/1 -> [F]
  [q] -> 2nd Order Filter Input ICs1/1(In)
  Product/1 -> x_dot/1
  OMNI Revised Kinematics/1(p) -> x/1
  [q] -> OMNI Revised Kinematics/1(M)
  q/1 -> [q]
  2nd Order Filter Input ICs1/2(Out_dot) -> Product/2
  OMNI Revised Kinematics/2(J) -> Product/1, J/1, [J]
  Constant6/1 -> 2nd Order Filter Input ICs1/3(z)
  Constant5/1 -> 2nd Order Filter Input ICs1/2(Wn)
  Constant2/1 -> OMNI Revised Kinematics/3(l2)
  Constant1/1 -> OMNI Revised Kinematics/2(l1)
  Constant3/1 -> OMNI Revised Kinematics/4(l3)
  2nd Order Filter Input ICs1/1(Out) -> Terminator_13/1

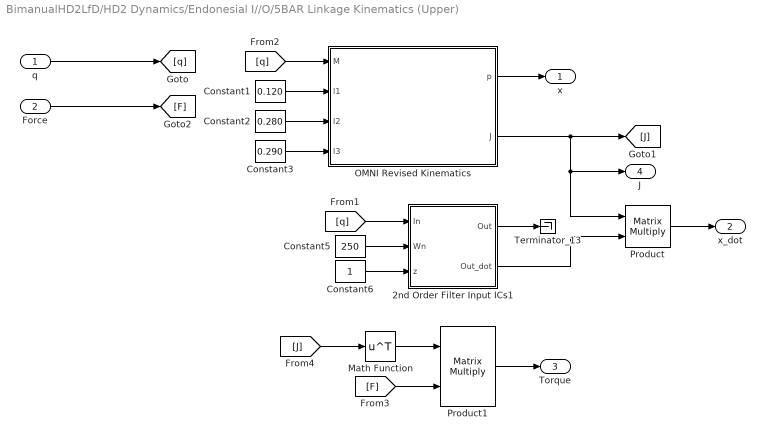
== system BimanualHD2LfD/HD2 Dynamics/Endonesial I//O/5BAR Linkage Kinematics (Upper) ==
  q : Inport
  Force : Inport  Port=2
  2nd Order Filter Input ICs1 : Subsystem
  Constant1 : Constant  Value=0.120
  Constant2 : Constant  Value=0.280
  Constant3 : Constant  Value=0.290
  Constant5 : Constant  Value=250
  Constant6 : Constant
  Math Function : Math  Operator=transpose  SaturateOnIntegerOverflow=on
  OMNI Revised Kinematics : MATLAB Function  TreatAsAtomicUnit=on
  Product : Product  Multiplication=Matrix(*)  RndMeth=Zero
  Product1 : Product  Multiplication=Matrix(*)  RndMeth=Zero
  Terminator_13 : Terminator
  x : Outport
  x_dot : Outport  Port=2
  Torque : Outport  Port=3
  J : Outport  Port=4
  wires:
  Math Function/1 -> Product1/1
  Product1/1 -> Torque/1
  [F] -> Product1/2
  [J] -> Math Function/1
  Force/1 -> [F]
  [q] -> 2nd Order Filter Input ICs1/1(In)
  Product/1 -> x_dot/1
  OMNI Revised Kinematics/1(p) -> x/1
  [q] -> OMNI Revised Kinematics/1(M)
  q/1 -> [q]
  2nd Order Filter Input ICs1/2(Out_dot) -> Product/2
  OMNI Revised Kinematics/2(J) -> Product/1, J/1, [J]
  Constant6/1 -> 2nd Order Filter Input ICs1/3(z)
  Constant5/1 -> 2nd Order Filter Input ICs1/2(Wn)
  Constant2/1 -> OMNI Revised Kinematics/3(l2)
  Constant1/1 -> OMNI Revised Kinematics/2(l1)
  Constant3/1 -> OMNI Revised Kinematics/4(l3)
  2nd Order Filter Input ICs1/1(Out) -> Terminator_13/1

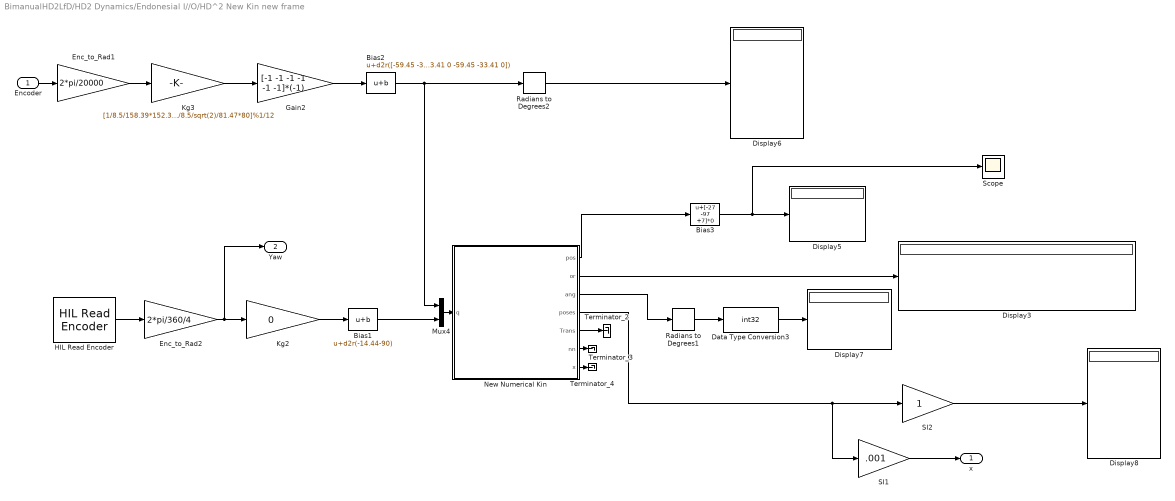
== system BimanualHD2LfD/HD2 Dynamics/Endonesial I//O/HD^2 New Kin new frame ==
  Encoder : Inport
  Bias1 : Bias  Bias=d2r(-14.44-90)
  Bias2 : Bias  Bias=d2r([-59.45 -33.41 0 -59.45 -33.41 0])
  Bias3 : Bias  Bias=[-27 -97 +7]*0
  Data Type Conversion3 : DataTypeConversion  OutDataTypeStr=int32
  Display{3,5..8} (5 alike) : Display
      Display3 settings: Decimation=1000
      Display5 settings: Decimation=1000
      Display6 settings: Decimation=1000
      Display7 settings: Decimation=100
      Display8 settings: Decimation=1000
  Enc_to_Rad1 : Gain  Gain=2*pi/20000
  Enc_to_Rad2 : Gain  Gain=2*pi/360/4
  Gain2 : Gain  Gain=[-1 -1 -1 -1 -1 -1]*(-1)
  HIL Read Encoder : quarc_library/Data Acquisition/Generic/Immediate I//O/HIL Read Encoder  object_name=HIL-1  channels=6  sample_time=qc_get_step_size  active=on  vector_output=off  data_type_mode=Inherit via back propagation  data_type=double
  Kg2 : Gain  Gain=0
  Kg3 : Gain  Gain=[1/8.5/158.39*152.34 1/8.5/156.47*152.34 1/8.5/sqrt(2)/40.6*40 1/8.5/159.39*152.34 1/8.5/154.97*152.34 1/8.5/sqrt(2)/81.47*80]%1/12
  Mux4 : Mux  Inputs=[6 1]
  New Numerical Kin : MATLAB Function  TreatAsAtomicUnit=on
  Radians to Degrees1 : simulink_extras/Transformations/Radians to Degrees
  Radians to Degrees2 : simulink_extras/Transformations/Radians to Degrees
  SI1 : Gain  Gain=.001
  SI2 : Gain
  Scope : Scope
  Terminator_2 : Terminator
  Terminator_3 : Terminator
  Terminator_4 : Terminator
  x : Outport
  Yaw : Outport  Port=2
  wires:
  New Numerical Kin/7(x) -> Terminator_4/1
  New Numerical Kin/6(nn) -> Terminator_3/1
  Mux4/1 -> New Numerical Kin/1(q)
  Bias1/1 -> Mux4/2
  Kg2/1 -> Bias1/1
  HIL Read Encoder/1 -> Enc_to_Rad2/1
  Enc_to_Rad2/1 -> Yaw/1, Kg2/1
  New Numerical Kin/5(Trans) -> Terminator_2/1
  New Numerical Kin/4(poses) -> SI1/1, SI2/1
  SI1/1 -> x/1
  Encoder/1 -> Enc_to_Rad1/1
  SI2/1 -> Display8/1
  New Numerical Kin/3(ang) -> Radians to Degrees1/1
  Data Type Conversion3/1 -> Display7/1
  Radians to Degrees1/1 -> Data Type Conversion3/1
  New Numerical Kin/2(or) -> Display3/1
  Bias3/1 -> Scope/1, Display5/1
  New Numerical Kin/1(pos) -> Bias3/1
  Radians to Degrees2/1 -> Display6/1
  Bias2/1 -> Mux4/1, Radians to Degrees2/1
  Kg3/1 -> Gain2/1
  Enc_to_Rad1/1 -> Kg3/1
  Gain2/1 -> Bias2/1

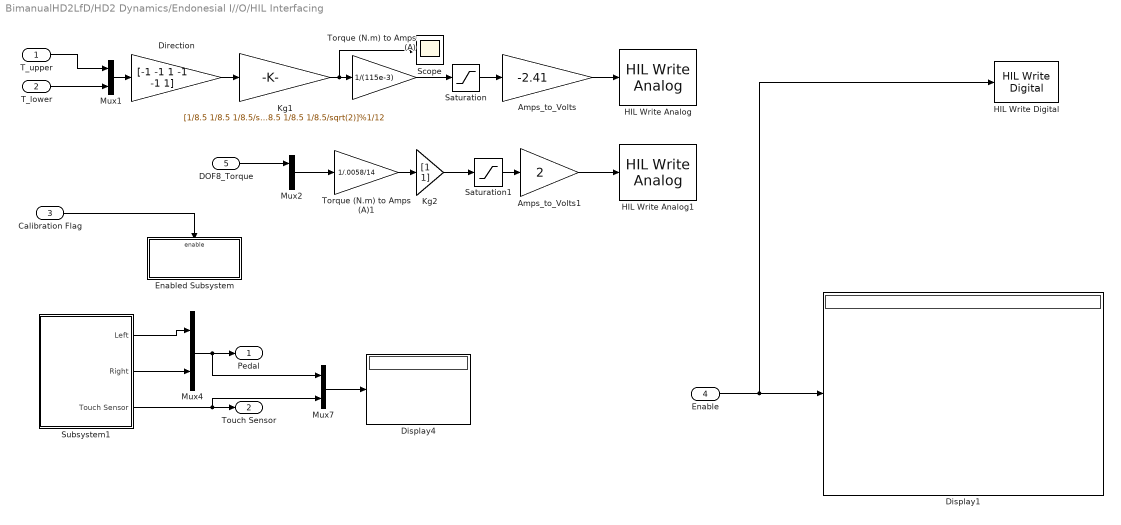
== system BimanualHD2LfD/HD2 Dynamics/Endonesial I//O/HIL Interfacing ==
  T_upper : Inport
  T_lower : Inport  Port=2
  Calibration Flag : Inport  Port=3
  Enable : Inport  Port=4
  DOF8_Torque : Inport  Port=5
  Amps_to_Volts : Gain  Gain=-2.41
  Amps_to_Volts1 : Gain  Gain=2
  Direction : Gain  Gain=[-1 -1 1 -1 -1 1]
  Display1 : Display
      settings: Decimation=100
  Display4 : Display
      settings: Decimation=100
  Enabled Subsystem : Subsystem  TreatAsAtomicUnit=on
  HIL Write Analog : quarc_library/Data Acquisition/Generic/Immediate I//O/HIL Write Analog  object_name=HIL-1  channels=0:5  sample_time=-1  active=off  vector_input=on
  HIL Write Analog1 : quarc_library/Data Acquisition/Generic/Immediate I//O/HIL Write Analog  object_name=HIL-1  channels=6:7  sample_time=-1  active=off  vector_input=on
  HIL Write Digital : quarc_library/Data Acquisition/Generic/Immediate I//O/HIL Write Digital  object_name=HIL-1  channels=9:10  sample_time=-1  active=off  vector_input=on
  Kg1 : Gain  Gain=[1/8.5 1/8.5 1/8.5/sqrt(2) 1/8.5 1/8.5 1/8.5/sqrt(2)]%1/12
  Kg2 : Gain  Gain=[1 1]
  Mux{1..2,4,7} (4 alike) : Mux  Inputs=2
  Saturation : Saturate  UpperLimit=5  LowerLimit=-5
  Saturation1 : Saturate  UpperLimit=.6  LowerLimit=-.6
  Scope : Scope
  Subsystem1 : Subsystem
  Torque (N.m) to Amps (A) : Gain  Gain=1/(115e-3)
  Torque (N.m) to Amps (A)1 : Gain  Gain=1/.0058/14
  Pedal : Outport
  "Touch Sensor " : Outport  Port=2
  wires:
  Torque (N.m) to Amps (A)1/1 -> Kg2/1
  Amps_to_Volts1/1 -> HIL Write Analog1/1
  Saturation1/1 -> Amps_to_Volts1/1
  Kg2/1 -> Saturation1/1
  Enable/1 -> HIL Write Digital/1, Display1/1
  Mux7/1 -> Display4/1
  Subsystem1/3(Touch Sensor) -> Mux7/2, "Touch Sensor "/1
  Mux4/1 -> Mux7/1, Pedal/1
  Subsystem1/2(Right) -> Mux4/2
  Subsystem1/1(Left) -> Mux4/1
  Calibration Flag/1 -> Enabled Subsystem/Enable
  T_upper/1 -> Mux1/1
  T_lower/1 -> Mux1/2
  Saturation/1 -> Amps_to_Volts/1
  Kg1/1 -> Torque (N.m) to Amps (A)/1, Scope/1
  Direction/1 -> Kg1/1
  Mux1/1 -> Direction/1
  Torque (N.m) to Amps (A)/1 -> Saturation/1
  Amps_to_Volts/1 -> HIL Write Analog/1
  Mux2/1 -> Torque (N.m) to Amps (A)1/1
  DOF8_Torque/1 -> Mux2/1

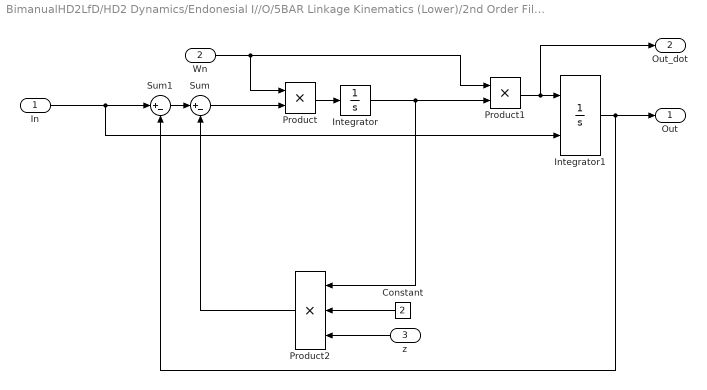
== system BimanualHD2LfD/HD2 Dynamics/Endonesial I//O/5BAR Linkage Kinematics (Lower)/2nd Order Filter Input ICs1 ==
  In : Inport
  Wn : Inport  Port=2
  z : Inport  Port=3
  Constant : Constant  Value=2
  Integrator : Integrator
  Integrator1 : Integrator  InitialConditionSource=external
  Product : Product  RndMeth=Zero
  Product1 : Product  RndMeth=Zero
  Product2 : Product  Inputs=3  RndMeth=Zero
  Sum : Sum  Inputs=|+-
  Sum1 : Sum  Inputs=|+-
  Out : Outport
  Out_dot : Outport  Port=2
  wires:
  Constant/1 -> Product2/2
  z/1 -> Product2/3
  Product2/1 -> Sum/2
  In/1 -> Integrator1/2, Sum1/1
  Sum1/1 -> Sum/1
  Integrator1/1 -> Out/1, Sum1/2
  Integrator/1 -> Product2/1, Product1/2
  Product1/1 -> Out_dot/1, Integrator1/1
  Wn/1 -> Product1/1, Product/1
  Sum/1 -> Product/2
  Product/1 -> Integrator/1

== system BimanualHD2LfD/HD2 Dynamics/Endonesial I//O/5BAR Linkage Kinematics (Upper)/2nd Order Filter Input ICs1 ==
  In : Inport
  Wn : Inport  Port=2
  z : Inport  Port=3
  Constant : Constant  Value=2
  Integrator : Integrator
  Integrator1 : Integrator  InitialConditionSource=external
  Product : Product  RndMeth=Zero
  Product1 : Product  RndMeth=Zero
  Product2 : Product  Inputs=3  RndMeth=Zero
  Sum : Sum  Inputs=|+-
  Sum1 : Sum  Inputs=|+-
  Out : Outport
  Out_dot : Outport  Port=2
  wires:
  Constant/1 -> Product2/2
  z/1 -> Product2/3
  Product2/1 -> Sum/2
  In/1 -> Integrator1/2, Sum1/1
  Sum1/1 -> Sum/1
  Integrator1/1 -> Out/1, Sum1/2
  Integrator/1 -> Product2/1, Product1/2
  Product1/1 -> Out_dot/1, Integrator1/1
  Wn/1 -> Product1/1, Product/1
  Sum/1 -> Product/2
  Product/1 -> Integrator/1

== system BimanualHD2LfD/HD2 Dynamics/Endonesial I//O/HIL Interfacing/Enabled Subsystem ==
  Enable : EnablePort
  HIL Set Encoder Counts : quarc_library/Data Acquisition/Generic/Configuration/HIL Set Encoder Counts  object_name=HIL-1  channels=[0:7]  source=internal  counts=0  sample_time=-1  active=on  vector_input=on
      settings: AttributesFormatString=(%<object_name>)

== system BimanualHD2LfD/HD2 Dynamics/Endonesial I//O/HIL Interfacing/Subsystem1 ==
  Constant2 : Constant  Value=0.01
  Data Type Conversion : DataTypeConversion
  Data Type Conversion1 : DataTypeConversion
  De Bouncer : Subsystem
  De Bouncer1 : Subsystem
  Display : Display
  Display1 : Display
  HIL Read Digital : quarc_library/Data Acquisition/Generic/Immediate I//O/HIL Read Digital  object_name=HIL-1  channels=[0 1 7]  sample_time=qc_get_step_size  active=on  vector_output=off  data_type_mode=Inherit via back propagation  data_type=boolean
      settings: AttributesFormatString=(%<object_name>)
  Left : Outport
  Right : Outport  Port=2
  Touch Sensor : Outport  Port=3
  wires:
  HIL Read Digital/3 -> Touch Sensor/1
  HIL Read Digital/2 -> Display/1, Data Type Conversion1/1
  HIL Read Digital/1 -> Display1/1, Data Type Conversion/1
  Data Type Conversion/1 -> De Bouncer/1(Input)
  Data Type Conversion1/1 -> De Bouncer1/1(Input)
  Constant2/1 -> De Bouncer1/2(debounce_time), De Bouncer/2(debounce_time)
  De Bouncer/1(Output) -> Left/1
  De Bouncer1/1(Output) -> Right/1

== system BimanualHD2LfD/HD2 Dynamics/Endonesial I//O/HIL Interfacing/Subsystem1/De Bouncer ==
  Input : Inport
  debounce_time : Inport  Port=2
  Data Type Conversion : DataTypeConversion  OutDataTypeStr=int32
  Embedded MATLAB Function : MATLAB Function  TreatAsAtomicUnit=on
  Gain : Gain  Gain=1/qc_get_step_size
  Memory : Memory  InheritSampleTime=on  LinearizeMemory=on  LinearizeAsDelay=on
  Memory1 : Memory  InheritSampleTime=on  LinearizeMemory=on  LinearizeAsDelay=on
  Output : Outport
  wires:
  Embedded MATLAB Function/1(output) -> Memory/1, Output/1
  Embedded MATLAB Function/2(counter) -> Memory1/1
  Memory/1 -> Embedded MATLAB Function/3(prev_output)
  Memory1/1 -> Embedded MATLAB Function/4(prev_counter)
  Input/1 -> Embedded MATLAB Function/1(input)
  debounce_time/1 -> Gain/1
  Data Type Conversion/1 -> Embedded MATLAB Function/2(num_samples)
  Gain/1 -> Data Type Conversion/1

== system BimanualHD2LfD/HD2 Dynamics/Endonesial I//O/HIL Interfacing/Subsystem1/De Bouncer1 ==
  Input : Inport
  debounce_time : Inport  Port=2
  Data Type Conversion : DataTypeConversion  OutDataTypeStr=int32
  Embedded MATLAB Function : MATLAB Function  TreatAsAtomicUnit=on
  Gain : Gain  Gain=1/qc_get_step_size
  Memory : Memory  InheritSampleTime=on  LinearizeMemory=on  LinearizeAsDelay=on
  Memory1 : Memory  InheritSampleTime=on  LinearizeMemory=on  LinearizeAsDelay=on
  Output : Outport
  wires:
  Gain/1 -> Data Type Conversion/1
  Data Type Conversion/1 -> Embedded MATLAB Function/2(num_samples)
  debounce_time/1 -> Gain/1
  Input/1 -> Embedded MATLAB Function/1(input)
  Memory1/1 -> Embedded MATLAB Function/4(prev_counter)
  Memory/1 -> Embedded MATLAB Function/3(prev_output)
  Embedded MATLAB Function/2(counter) -> Memory1/1
  Embedded MATLAB Function/1(output) -> Output/1, Memory/1

== matlab function BimanualHD2LfD/GMR/MATLAB Function ==
  data: outputs output; data input; I_vars input; O_vars input; output_var output; model parameter
function [outputs, output_var] = GMR_3DOF (data, I_vars, O_vars, model) 
%#codegen
    [outputs, output_var, ~] = GMR(model, data, I_vars, O_vars);
end

== matlab function BimanualHD2LfD/Remove Orientation Jump/Remove Orientation Jump ==
  data: signal input; prevSignal input; out output; time input
function out = removeJump(signal, prevSignal, time)
persistent jumpType;
persistent jumpDistance;
persistent jumpCounter;


    if isempty(jumpType) || (time < 0.1)
        jumpType = 0;
        jumpDistance = 0;
        jumpCounter = 0;
    end

    if (signal - prevSignal) < -1
        jumpType = -1;
        jumpCounter = jumpCounter - 1;
        jumpDistance = signal-prevSignal;
        
    elseif (signal - prevSignal) > 1
        jumpType = 1;
        jumpCounter = jumpCounter + 1;
        jumpDistance = signal-prevSignal;
    end
    
    if jumpType == 1
        out = signal - jumpDistance*jumpCounter;
    elseif jumpType == -1
        out = signal + jumpDistance*jumpCounter;
    else
        out = signal;
    end
end
